simulink model "vel_testing"  (R2018b)
settings: Solver=FixedStepAuto  StartTime=0.0  StopTime=13  FixedStep=continuous_h  RelTol=1e-3
StopFcn:
  | res_vel_test = process_vel_testing(vel_state, vel_ref);
libraries: simulink x3, cf_lib x1, vel_controller_lib x1
settings Model: Creator=sebbe  LastModifiedBy=Pontus

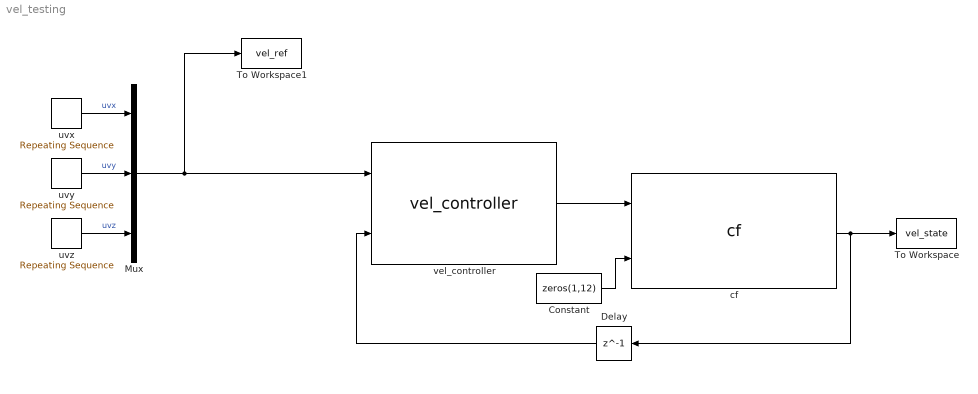
== system vel_testing ==
  Constant : Constant  Value=zeros(1,12)
  Delay : Delay  DelayLength=1
  Mux : Mux  Inputs=3
  To Workspace : ToWorkspace  VariableName=vel_state  SaveFormat=Timeseries  SampleTime=-1
  To Workspace1 : ToWorkspace  VariableName=vel_ref  SaveFormat=Timeseries  SampleTime=-1
  cf : cf_lib/cf  SystemSampleTime=-1
  uvx : simulink/Sources/Repeating Sequence  rep_seq_t=time_ref  rep_seq_y=ref.x
  uvy : simulink/Sources/Repeating Sequence  rep_seq_t=time_ref  rep_seq_y=ref.y
  uvz : simulink/Sources/Repeating Sequence  rep_seq_t=time_ref  rep_seq_y=ref.z
  vel_controller : vel_controller_lib/vel_controller  SystemSampleTime=-1
  wires:
  uvx/1 -> Mux/1  "uvx"
  uvy/1 -> Mux/2  "uvy"
  uvz/1 -> Mux/3  "uvz"
  Mux/1 -> vel_controller/1, To Workspace1/1
  vel_controller/1 -> cf/1
  Constant/1 -> cf/2
  cf/1 -> To Workspace/1, Delay/1
  Delay/1 -> vel_controller/2
